simulink model "sualai"  (R2015a)
settings: Solver=ode45  StartTime=0.0  StopTime=10.0  RelTol=1e-3
undefined symbols (not defined in the file or in its folder): Khau4, RBS, RootGround, RootPart, sualai
libraries: mblibv1 x14
settings Model: Creator=Administrator  LastModifiedBy=Administrator
settings SimMechanicsCC: VisOnUpdateDiagram=on  VisDuringSimulation=on

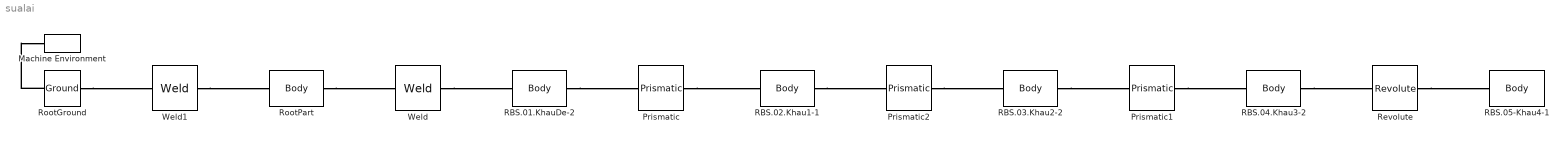
== system sualai ==
  Machine Environment : mblibv1/Bodies/Machine Environment  PortType=env  PhysicalDomain=Mechanical  DialogTemplateClass=MECH.MachineEnvironment  SyncWhenCopied=off  Gravity=[0 -9.81 0]  GravityUnits=m/s^2  GravityAsSignal=off  Dimensionality=Auto-detect  AnalysisType=Forward dynamics  LinearAssemblyTolerance=1e-3  LinearAssemblyToleranceUnits=m  AngularAssemblyTolerance=1e-3  AngularAssemblyToleranceUnits=rad  ConstraintSolverType=Stabilizing  ConstraintRelTolerance=1e-4  ConstraintAbsTolerance=1e-4  UseRobustSingularityHandling=off  RedundancyAnalysisToleranceType=Automatically select tolerance  RedundancyAnalysisTolerance=1e-14  StatePerturbationType=Fixed  PerturbationSize=1e-5  VisualizeMachine=on  BodyVisualizationType=Use model default body geometries  BodyColorSelMode=Use model default  DefaultBodyColor=[1 0 0]
  Prismatic : mblibv1/Joints/Prismatic  LConnTagsString=__newl0  RConnTagsString=__newr0  UpdateFromCAD=on  PMImportedID=RBS.01.KhauDe-2:-:RBS.02.Khau1-1  NumSAPorts=0  CutJoint=off  MarkAsCut=off  Primitives=prismatic  PrimitiveProps=P1$WORLD$[0,0,1]$prismatic  DialogClass=JointBlock  P1Axis=[0,0,1]
  Prismatic1 : mblibv1/Joints/Prismatic  LConnTagsString=__newl0  RConnTagsString=__newr0  UpdateFromCAD=on  PMImportedID=RBS.03.Khau2-2:-:RBS.04.Khau3-2  NumSAPorts=0  CutJoint=off  MarkAsCut=off  Primitives=prismatic  PrimitiveProps=P1$WORLD$[0,-1,0]$prismatic  DialogClass=JointBlock  P1Axis=[0,-1,0]
  Prismatic2 : mblibv1/Joints/Prismatic  LConnTagsString=__newl0  RConnTagsString=__newr0  UpdateFromCAD=on  PMImportedID=RBS.02.Khau1-1:-:RBS.03.Khau2-2  NumSAPorts=0  CutJoint=off  MarkAsCut=off  Primitives=prismatic  PrimitiveProps=P1$WORLD$[-1,0,0]$prismatic  DialogClass=JointBlock  P1Axis=[-1,0,0]
  RBS.01.KhauDe-2 : mblibv1/Bodies/Body  LConnTagsString=CS2  RConnTagsString=CS3  UpdateFromCAD=on  PMImportedID=RBS.01.KhauDe-2  DialogClass=MechanicalBodyBlock  Mass=0.481266  MassUnits=kg  InertiaUnits=kg*m^2  Inertia=[3.26313,0,0;0,3.76071,0;0,0,1.18222]  Shape=Cylinder  ShapeDims=[1 1]  ShapeUnits=m  ShapeUse=false  Density=1  DensityUnits=kg/m^3  DensityUse=false  GraphicsMode=GFXFILE  GraphicsFileName=sualai - RBS.01.KhauDe-2.STL  BodyColorSelMode=COLORPALETTE  BodyColor=[0.65098;0.619608;0.588235]  AttachedToCS=CS1  CG=Right$CG$[1.35 0.730871 2.35]$WORLD$WORLD$m$[1 0 0;0 1 0;0 0 1]$3x3 Transform$rad$WORLD$false$RBS.01.KhauDe-2::CG(AUTOGEN)  WorkingFrames=Right$CS1$[0 0 0]$WORLD$WORLD$m$[1 0 0;0 1 0;0 0 1]$3x3 Transform$rad$WORLD$false$RBS.01.KhauDe-2::CS1(AUTOGEN)#Left$CS2$[1.35 0.730871 2.35]$WORLD$WORLD$m$[1 0 0;0 1 0;0 0 1]$3x3 Transform$rad$WORLD$true$RBS.01.KhauDe-2:-:sualai/RootPart::RBS.01.KhauDe-2(AUTOGEN)#Right$CS3$[0.283311 0.05 2.89491]$WORLD$WORLD$m$[1 0 0;0 1 0;0 0 1]$3x3 Transform$rad$WORLD$true$RBS.01.KhauDe-2:-:RBS.02.Khau1-1::RBS.01.KhauDe-2(AUTOGEN)  CGPos=[1.35 0.730871 2.35]  CGRot=[1 0 0;0 1 0;0 0 1]  CS0Pos=[]  CS0Rot=[]  CS1Pos=[0 0 0]  CS1Rot=[1 0 0;0 1 0;0 0 1]  CS2Pos=[1.35 0.730871 2.35]  CS2Rot=[1 0 0;0 1 0;0 0 1]  CS3Pos=[0.283311 0.05 2.89491]  CS3Rot=[1 0 0;0 1 0;0 0 1]  CS4Pos=[]  CS4Rot=[]  CS5Pos=[]  CS5Rot=[]  CS6Pos=[]  CS6Rot=[]  CS7Pos=[]  CS7Rot=[]  CS8Pos=[]  CS8Rot=[]  CS9Pos=[]  CS9Rot=[]  CS10Pos=[]  CS10Rot=[]  CS11Pos=[]  CS11Rot=[]  CS12Pos=[]  CS12Rot=[]  CS13Pos=[]  CS13Rot=[]  CS14Pos=[]  CS14Rot=[]  CS15Pos=[]  CS15Rot=[]  CS16Pos=[]  CS16Rot=[]  CS17Pos=[]  CS17Rot=[]  CS18Pos=[]  CS18Rot=[]  CS19Pos=[]  CS19Rot=[]  CS20Pos=[]  CS20Rot=[]
  RBS.02.Khau1-1 : mblibv1/Bodies/Body  LConnTagsString=CS2  RConnTagsString=CS3  UpdateFromCAD=on  PMImportedID=RBS.02.Khau1-1  DialogClass=MechanicalBodyBlock  Mass=0.091  MassUnits=kg  InertiaUnits=kg*m^2  Inertia=[0.0767067,0,0;0,0.0683701,0;0,0,0.00850512]  Shape=Cylinder  ShapeDims=[1 1]  ShapeUnits=m  ShapeUse=false  Density=1  DensityUnits=kg/m^3  DensityUse=false  GraphicsMode=GFXFILE  GraphicsFileName=sualai - RBS.02.Khau1-1.STL  BodyColorSelMode=COLORPALETTE  BodyColor=[0.65098;0.619608;0.588235]  AttachedToCS=CS1  CG=Right$CG$[1.35 -0.0387363 -0.1]$WORLD$WORLD$m$[0 0 1;-1 0 0;0 -1 0]$3x3 Transform$rad$WORLD$false$RBS.02.Khau1-1::CG(AUTOGEN)  WorkingFrames=Right$CS1$[0.2 -0.1 -0.1]$WORLD$WORLD$m$[0 0 1;-1 0 0;0 -1 0]$3x3 Transform$rad$WORLD$false$RBS.02.Khau1-1::CS1(AUTOGEN)#Left$CS2$[0.283311 0.05 2.89491]$WORLD$WORLD$m$[1 0 0;0 1 0;0 0 1]$3x3 Transform$rad$WORLD$true$RBS.01.KhauDe-2:-:RBS.02.Khau1-1::RBS.02.Khau1-1(AUTOGEN)#Right$CS3$[0.692403 -0.1 -0.471467]$WORLD$WORLD$m$[1 0 0;0 1 0;0 0 1]$3x3 Transform$rad$WORLD$true$RBS.02.Khau1-1:-:RBS.03.Khau2-2::RBS.02.Khau1-1(AUTOGEN)  CGPos=[1.35 -0.0387363 -0.1]  CGRot=[0 0 1;-1 0 0;0 -1 0]  CS0Pos=[]  CS0Rot=[]  CS1Pos=[0.2 -0.1 -0.1]  CS1Rot=[0 0 1;-1 0 0;0 -1 0]  CS2Pos=[0.283311 0.05 2.89491]  CS2Rot=[1 0 0;0 1 0;0 0 1]  CS3Pos=[0.692403 -0.1 -0.471467]  CS3Rot=[1 0 0;0 1 0;0 0 1]  CS4Pos=[]  CS4Rot=[]  CS5Pos=[]  CS5Rot=[]  CS6Pos=[]  CS6Rot=[]  CS7Pos=[]  CS7Rot=[]  CS8Pos=[]  CS8Rot=[]  CS9Pos=[]  CS9Rot=[]  CS10Pos=[]  CS10Rot=[]  CS11Pos=[]  CS11Rot=[]  CS12Pos=[]  CS12Rot=[]  CS13Pos=[]  CS13Rot=[]  CS14Pos=[]  CS14Rot=[]  CS15Pos=[]  CS15Rot=[]  CS16Pos=[]  CS16Rot=[]  CS17Pos=[]  CS17Rot=[]  CS18Pos=[]  CS18Rot=[]  CS19Pos=[]  CS19Rot=[]  CS20Pos=[]  CS20Rot=[]
  RBS.03.Khau2-2 : mblibv1/Bodies/Body  LConnTagsString=CS3  RConnTagsString=CS2  UpdateFromCAD=on  PMImportedID=RBS.03.Khau2-2  DialogClass=MechanicalBodyBlock  Mass=678.24  MassUnits=kg  InertiaUnits=kg*m^2  Inertia=[193.644,0,0;0,196.51,-6.39404;0,-6.39404,12.4099]  Shape=Cylinder  ShapeDims=[1 1]  ShapeUnits=m  ShapeUse=false  Density=1  DensityUnits=kg/m^3  DensityUse=false  GraphicsMode=GFXFILE  GraphicsFileName=sualai - RBS.03.Khau2-2.STL  BodyColorSelMode=COLORPALETTE  BodyColor=[1;0;0]  AttachedToCS=CS1  CG=Right$CG$[0.213657 -0.135278 -0.1]$WORLD$WORLD$m$[0 1 0;0 0 1;1 0 0]$3x3 Transform$rad$WORLD$false$RBS.03.Khau2-2::CG(AUTOGEN)  WorkingFrames=Right$CS1$[0.4 -1.09 -0.1]$WORLD$WORLD$m$[0 1 0;0 0 1;1 0 0]$3x3 Transform$rad$WORLD$false$RBS.03.Khau2-2::CS1(AUTOGEN)#Right$CS2$[0.340796 -0.618126 -0.2]$WORLD$WORLD$m$[1 0 0;0 1 0;0 0 1]$3x3 Transform$rad$WORLD$true$RBS.03.Khau2-2:-:RBS.04.Khau3-2::RBS.03.Khau2-2(AUTOGEN)#Left$CS3$[0.692403 -0.1 -0.471467]$WORLD$WORLD$m$[1 0 0;0 1 0;0 0 1]$3x3 Transform$rad$WORLD$true$RBS.02.Khau1-1:-:RBS.03.Khau2-2::RBS.03.Khau2-2(AUTOGEN)  CGPos=[0.213657 -0.135278 -0.1]  CGRot=[0 1 0;0 0 1;1 0 0]  CS0Pos=[]  CS0Rot=[]  CS1Pos=[0.4 -1.09 -0.1]  CS1Rot=[0 1 0;0 0 1;1 0 0]  CS2Pos=[0.340796 -0.618126 -0.2]  CS2Rot=[1 0 0;0 1 0;0 0 1]  CS3Pos=[0.692403 -0.1 -0.471467]  CS3Rot=[1 0 0;0 1 0;0 0 1]  CS4Pos=[]  CS4Rot=[]  CS5Pos=[]  CS5Rot=[]  CS6Pos=[]  CS6Rot=[]  CS7Pos=[]  CS7Rot=[]  CS8Pos=[]  CS8Rot=[]  CS9Pos=[]  CS9Rot=[]  CS10Pos=[]  CS10Rot=[]  CS11Pos=[]  CS11Rot=[]  CS12Pos=[]  CS12Rot=[]  CS13Pos=[]  CS13Rot=[]  CS14Pos=[]  CS14Rot=[]  CS15Pos=[]  CS15Rot=[]  CS16Pos=[]  CS16Rot=[]  CS17Pos=[]  CS17Rot=[]  CS18Pos=[]  CS18Rot=[]  CS19Pos=[]  CS19Rot=[]  CS20Pos=[]  CS20Rot=[]
  RBS.04.Khau3-2 : mblibv1/Bodies/Body  LConnTagsString=CS3  RConnTagsString=CS2  UpdateFromCAD=on  PMImportedID=RBS.04.Khau3-2  DialogClass=MechanicalBodyBlock  Mass=368.144  MassUnits=kg  InertiaUnits=kg*m^2  Inertia=[112.705,0,0;0,112.705,0;0,0,3.324]  Shape=Cylinder  ShapeDims=[1 1]  ShapeUnits=m  ShapeUse=false  Density=1  DensityUnits=kg/m^3  DensityUse=false  GraphicsMode=GFXFILE  GraphicsFileName=sualai - RBS.04.Khau3-2.STL  BodyColorSelMode=COLORPALETTE  BodyColor=[0;1;1]  AttachedToCS=CS1  CG=Right$CG$[0.4 -0.137732 -0.1]$WORLD$WORLD$m$[0 1 0;0 0 1;1 0 0]$3x3 Transform$rad$WORLD$false$RBS.04.Khau3-2::CG(AUTOGEN)  WorkingFrames=Right$CS1$[0.4 0.71 -0.1]$WORLD$WORLD$m$[0 1 0;0 0 1;1 0 0]$3x3 Transform$rad$WORLD$false$RBS.04.Khau3-2::CS1(AUTOGEN)#Right$CS2$[0.4 0.71 -0.1]$WORLD$WORLD$m$[1 0 0;0 1 0;0 0 1]$3x3 Transform$rad$WORLD$true$RBS.04.Khau3-2:-:RBS.05-Khau4-1::RBS.04.Khau3-2(AUTOGEN)#Left$CS3$[0.340796 -0.618126 -0.2]$WORLD$WORLD$m$[1 0 0;0 1 0;0 0 1]$3x3 Transform$rad$WORLD$true$RBS.03.Khau2-2:-:RBS.04.Khau3-2::RBS.04.Khau3-2(AUTOGEN)  CGPos=[0.4 -0.137732 -0.1]  CGRot=[0 1 0;0 0 1;1 0 0]  CS0Pos=[]  CS0Rot=[]  CS1Pos=[0.4 0.71 -0.1]  CS1Rot=[0 1 0;0 0 1;1 0 0]  CS2Pos=[0.4 0.71 -0.1]  CS2Rot=[1 0 0;0 1 0;0 0 1]  CS3Pos=[0.340796 -0.618126 -0.2]  CS3Rot=[1 0 0;0 1 0;0 0 1]  CS4Pos=[]  CS4Rot=[]  CS5Pos=[]  CS5Rot=[]  CS6Pos=[]  CS6Rot=[]  CS7Pos=[]  CS7Rot=[]  CS8Pos=[]  CS8Rot=[]  CS9Pos=[]  CS9Rot=[]  CS10Pos=[]  CS10Rot=[]  CS11Pos=[]  CS11Rot=[]  CS12Pos=[]  CS12Rot=[]  CS13Pos=[]  CS13Rot=[]  CS14Pos=[]  CS14Rot=[]  CS15Pos=[]  CS15Rot=[]  CS16Pos=[]  CS16Rot=[]  CS17Pos=[]  CS17Rot=[]  CS18Pos=[]  CS18Rot=[]  CS19Pos=[]  CS19Rot=[]  CS20Pos=[]  CS20Rot=[]
  RBS.05-Khau4-1 : mblibv1/Bodies/Body  LConnTagsString=CS2  UpdateFromCAD=on  PMImportedID=RBS.05-Khau4-1  DialogClass=MechanicalBodyBlock  Mass=26.144  MassUnits=kg  InertiaUnits=kg*m^2  Inertia=[0.122087,0,0;0,0.139242,0;0,0,0.219027]  Shape=Cylinder  ShapeDims=[1 1]  ShapeUnits=m  ShapeUse=false  Density=1  DensityUnits=kg/m^3  DensityUse=false  GraphicsMode=GFXFILE  GraphicsFileName=sualai - RBS.05-Khau4-1.STL  BodyColorSelMode=COLORPALETTE  BodyColor=[1;1;0]  AttachedToCS=CS1  CG=Right$CG$[0.399939 0.76 -0.0952544]$WORLD$WORLD$m$[-0.0129085 0.999917 0;0 0 1;0.999917 0.0129085 0]$3x3 Transform$rad$WORLD$false$RBS.05-Khau4-1::CG(AUTOGEN)  WorkingFrames=Right$CS1$[0.396773 0.76 0.149979]$WORLD$WORLD$m$[-0.0129085 0.999917 0;0 0 1;0.999917 0.0129085 0]$3x3 Transform$rad$WORLD$false$RBS.05-Khau4-1::CS1(AUTOGEN)#Left$CS2$[0.4 0.71 -0.1]$WORLD$WORLD$m$[1 0 0;0 1 0;0 0 1]$3x3 Transform$rad$WORLD$true$RBS.04.Khau3-2:-:RBS.05-Khau4-1::RBS.05-Khau4-1(AUTOGEN)  CGPos=[0.399939 0.76 -0.0952544]  CGRot=[-0.0129085 0.999917 0;0 0 1;0.999917 0.0129085 0]  CS0Pos=[]  CS0Rot=[]  CS1Pos=[0.396773 0.76 0.149979]  CS1Rot=[-0.0129085 0.999917 0;0 0 1;0.999917 0.0129085 0]  CS2Pos=[0.4 0.71 -0.1]  CS2Rot=[1 0 0;0 1 0;0 0 1]  CS3Pos=[]  CS3Rot=[]  CS4Pos=[]  CS4Rot=[]  CS5Pos=[]  CS5Rot=[]  CS6Pos=[]  CS6Rot=[]  CS7Pos=[]  CS7Rot=[]  CS8Pos=[]  CS8Rot=[]  CS9Pos=[]  CS9Rot=[]  CS10Pos=[]  CS10Rot=[]  CS11Pos=[]  CS11Rot=[]  CS12Pos=[]  CS12Rot=[]  CS13Pos=[]  CS13Rot=[]  CS14Pos=[]  CS14Rot=[]  CS15Pos=[]  CS15Rot=[]  CS16Pos=[]  CS16Rot=[]  CS17Pos=[]  CS17Rot=[]  CS18Pos=[]  CS18Rot=[]  CS19Pos=[]  CS19Rot=[]  CS20Pos=[]  CS20Rot=[]
  Revolute : mblibv1/Joints/Revolute  LConnTagsString=__newl0  RConnTagsString=__newr0  UpdateFromCAD=on  PMImportedID=RBS.04.Khau3-2:-:RBS.05-Khau4-1  NumSAPorts=0  CutJoint=off  MarkAsCut=off  Primitives=prismatic  PrimitiveProps=R1$WORLD$[0,1,0]$revolute  DialogClass=JointBlock  R1Axis=[0,1,0]
  RootGround : mblibv1/Bodies/Ground  UpdateFromCAD=on  PMImportedID=RootGround  LeftPortType=env  RightPortType=workingframe  PhysicalDomain=Mechanical  DialogClass=GroundBlock  CoordPosition=[1.14419,0.469185,1.56332]  CoordPositionUnits=m  StateVectorMgrId=1  MachineId=[2 0]  ShowEnvPort=on  ParameterChecksum=[2537667724, 1906774507, 1690828522, 558254702]  TopologyChecksum=[892152192, 2153372925, 310781253, 957395988]
  RootPart : mblibv1/Bodies/Body  LConnTagsString=CS3  RConnTagsString=CS2  UpdateFromCAD=on  PMImportedID=sualai/RootPart  DialogClass=MechanicalBodyBlock  Mass=0  MassUnits=kg  InertiaUnits=kg*m^2  Inertia=[0,0,0;0,0,0;0,0,0]  Shape=Cylinder  ShapeDims=[1 1]  ShapeUnits=m  ShapeUse=false  Density=1  DensityUnits=kg/m^3  DensityUse=false  GraphicsMode=MACHINE_DEFAULT  BodyColorSelMode=MACHINE_DEFAULT  BodyColor=[1;0;0]  AttachedToCS=CS1  CG=Right$CG$[1.14419 0.469185 1.56332]$WORLD$WORLD$m$[1 0 0;0 1 0;0 0 1]$3x3 Transform$rad$WORLD$false$sualai/RootPart::CG(AUTOGEN)  WorkingFrames=Right$CS1$[0 0 0]$WORLD$WORLD$m$[1 0 0;0 1 0;0 0 1]$3x3 Transform$rad$WORLD$false$sualai/RootPart::CS1(AUTOGEN)#Right$CS2$[1.35 0.730871 2.35]$WORLD$WORLD$m$[1 0 0;0 1 0;0 0 1]$3x3 Transform$rad$WORLD$true$RBS.01.KhauDe-2:-:sualai/RootPart::sualai/RootPart(AUTOGEN)#Left$CS3$[1.14419 0.469185 1.56332]$WORLD$WORLD$m$[1 0 0;0 1 0;0 0 1]$3x3 Transform$rad$WORLD$true$RootGround:-:sualai/RootPart::sualai/RootPart(AUTOGEN)  CGPos=[1.14419 0.469185 1.56332]  CGRot=[1 0 0;0 1 0;0 0 1]  CS0Pos=[]  CS0Rot=[]  CS1Pos=[0 0 0]  CS1Rot=[1 0 0;0 1 0;0 0 1]  CS2Pos=[1.35 0.730871 2.35]  CS2Rot=[1 0 0;0 1 0;0 0 1]  CS3Pos=[1.14419 0.469185 1.56332]  CS3Rot=[1 0 0;0 1 0;0 0 1]  CS4Pos=[]  CS4Rot=[]  CS5Pos=[]  CS5Rot=[]  CS6Pos=[]  CS6Rot=[]  CS7Pos=[]  CS7Rot=[]  CS8Pos=[]  CS8Rot=[]  CS9Pos=[]  CS9Rot=[]  CS10Pos=[]  CS10Rot=[]  CS11Pos=[]  CS11Rot=[]  CS12Pos=[]  CS12Rot=[]  CS13Pos=[]  CS13Rot=[]  CS14Pos=[]  CS14Rot=[]  CS15Pos=[]  CS15Rot=[]  CS16Pos=[]  CS16Rot=[]  CS17Pos=[]  CS17Rot=[]  CS18Pos=[]  CS18Rot=[]  CS19Pos=[]  CS19Rot=[]  CS20Pos=[]  CS20Rot=[]
  Weld : mblibv1/Joints/Weld  LConnTagsString=__newl0  RConnTagsString=__newr0  UpdateFromCAD=on  PMImportedID=RBS.01.KhauDe-2:-:sualai/RootPart  NumSAPorts=0  CutJoint=off  MarkAsCut=off  Primitives=weld  PrimitiveProps=W$WORLD$[0.57735,0.57735,0.57735]$weld  DialogClass=JointBlock  WAxis=[0.57735,0.57735,0.57735]
  Weld1 : mblibv1/Joints/Weld  LConnTagsString=__newl0  RConnTagsString=__newr0  UpdateFromCAD=on  PMImportedID=RootGround:-:sualai/RootPart  NumSAPorts=0  CutJoint=off  MarkAsCut=off  Primitives=weld  PrimitiveProps=W$WORLD$[0.57735,0.57735,0.57735]$weld  DialogClass=JointBlock  WAxis=[0.57735,0.57735,0.57735]
  connections:
  RootPart/RConn1 -- Weld/LConn1
  Weld/RConn1 -- RBS.01.KhauDe-2/LConn1
  RBS.01.KhauDe-2/RConn1 -- Prismatic/LConn1
  Prismatic/RConn1 -- RBS.02.Khau1-1/LConn1
  RBS.04.Khau3-2/RConn1 -- Revolute/LConn1
  Revolute/RConn1 -- RBS.05-Khau4-1/LConn1
  RBS.03.Khau2-2/RConn1 -- Prismatic1/LConn1
  Prismatic1/RConn1 -- RBS.04.Khau3-2/LConn1
  RBS.02.Khau1-1/RConn1 -- Prismatic2/LConn1
  Prismatic2/RConn1 -- RBS.03.Khau2-2/LConn1
  RootGround/RConn1 -- Weld1/LConn1
  Weld1/RConn1 -- RootPart/LConn1
  RootGround/LConn1 -- Machine Environment/RConn1
